simulink model "sim_dist_pos_obs_paper"  (R2020a)
settings: Solver=ode4  StartTime=0.0  StopTime=30.0  FixedStep=0.01  RelTol=1e-3
values from neighbouring files (symbols this model uses):
  alfa_theta = 20    [draw_compare_dist_pos_obs.m]
  alfa_theta_obs = 100    [draw_compare_dist_pos_obs.m]
  beta1 = 1.2    [draw_compare_dist_pos_obs.m]
  beta2 = 0.8    [draw_compare_dist_pos_obs.m]
  c1_diff_sigma_bar_v = diag([25; 30; 20])    [draw_compare_dist_pos_obs.m]
  c1v = diag([16.0; 16.0; 16.0])    [draw_compare_dist_pos_obs.m]
  c2_diff_sigma_bar_v = diag([50; 50; 10])    [draw_compare_dist_pos_obs.m]
  c2v = diag([16.0; 16.0; 16.0])    [draw_compare_dist_pos_obs.m]
  c3_diff_sigma_bar_v = diag([15; 15; 10])    [draw_compare_dist_pos_obs.m]
  c3v = diag([16.0; 16.0; 16.0])    [draw_compare_dist_pos_obs.m]
  delta_p_i_0 = zeros(3, NF)    [draw_compare_dist_pos_obs.m]
  delta_v_i_0 = zeros(3, NF)    [draw_compare_dist_pos_obs.m]
  dp_aa_t = 0.2 * ones(3, 5) + ( 1.0 - 0.2 ) * rand(3, 5)    [draw_compare_dist_pos_obs.m]
  dp_ff_t = [ 0.4 * ones(1, 5) + ( 1.0 - 0.4 ) * rand(1, 5);                      0.4 * ones(1, 5) + ( 1.0 - 0.4 ) * rand(1, 5);                      0.2 * ones(1, 5) + ( 0.6 - 0.2 ) * rand(1, 5) ]    [draw_compare_dist_pos_obs.m]
  dp_phi_t = ( - pi / 2 ) * ones(3, 5) + ( pi / 2 - ( - pi / 2 ) ) * rand(3, 5)    [draw_compare_dist_pos_obs.m]
  etai_0 = zeros(3,5)    [draw_compare_dist_pos_obs.m]
  kai_1_t = 0.02    [draw_compare_dist_pos_obs.m]
  kai_3_t = 0.1    [draw_compare_dist_pos_obs.m]
  kai_chi_1 = diag([6; 6; 6])    [draw_compare_dist_pos_obs.m]
  kai_chi_2 = diag([6; 6; 6])    [draw_compare_dist_pos_obs.m]
  kai_u_1 = diag([8; 8; 8])    [draw_compare_dist_pos_obs.m]
  kai_u_2 = diag([8; 8; 8])    [draw_compare_dist_pos_obs.m]
  ksii_0 = zeros(3,5)    [draw_compare_dist_pos_obs.m]
  l1v = diag([20; 20; 20])    [draw_compare_dist_pos_obs.m]
  l2v = diag([30; 30; 30])    [draw_compare_dist_pos_obs.m]
  Lamd_diff_sigma_bar_v = 0.5    [draw_compare_dist_pos_obs.m]
  mass_i = zeros(1,NF)    [draw_compare_dist_pos_obs.m]
  Mii = diag([1;0;0;0;1])    [draw_compare_dist_pos_obs.m]
  pos0 = zeros(3, 1)    [draw_compare_dist_pos_obs.m]
  PZ0 = P0(3)    [draw_compare_dist_pos_obs.m]
  PZ1 = 10    [draw_compare_dist_pos_obs.m]
  Qci_init = repmat([1;0;0;0],1,NF)    [draw_compare_dist_pos_obs.m]
  R0 = 4    [draw_compare_dist_pos_obs.m]
  R1 = 8    [draw_compare_dist_pos_obs.m]
  Rx2 = 10    [draw_compare_dist_pos_obs.m]
  Ry2 = 6    [draw_compare_dist_pos_obs.m]
  Rz2 = 4    [draw_compare_dist_pos_obs.m]
  T0 = 0    [draw_compare_dist_pos_obs.m]
  T1 = tseq1    (= 10)    [draw_compare_dist_pos_obs.m]
  T12 = tseq1 + tseq12    (= 20)    [draw_compare_dist_pos_obs.m]
  T2 = tseq1 + tseq12 + tseq2    (= 30)    [draw_compare_dist_pos_obs.m]
  theta0 = ( 2 / 5 ) * pi    (= 1.25663706144)    [draw_compare_dist_pos_obs.m]
  vel0 = zeros(3, 1)    [draw_compare_dist_pos_obs.m]
  Wij = [0,0,1,0,0;              0,0,1,1,0;              1,0,0,0,1;              0,1,1,0,0;              0,0,1,0,0]    [draw_compare_dist_pos_obs.m]
  X1 = 8    [draw_compare_dist_pos_obs.m]
  X2 = 2    [draw_compare_dist_pos_obs.m]
  X3 = 3    [draw_compare_dist_pos_obs.m]
  Y1 = 10    [draw_compare_dist_pos_obs.m]
  Y2 = 2    [draw_compare_dist_pos_obs.m]
  Y3 = 4    [draw_compare_dist_pos_obs.m]
  Z1 = 4    [draw_compare_dist_pos_obs.m]
  Z2 = -6    [draw_compare_dist_pos_obs.m]
  Z3 = 2    [draw_compare_dist_pos_obs.m]
  zeta_diff_sigma_bar_v = 0.08    [draw_compare_dist_pos_obs.m]
undefined symbols (not defined in the file or in its folder): cal_frac_squ, p_alfav1, p_alfav2, p_beta1, p_beta2, p_dbeta1, p_dbeta2, p_gamma1_pos, p_gamma1_vel, p_gamma2_pos, p_gamma2_vel, q_alfav1, q_alfav2, q_beta1, q_beta2, q_dbeta1, q_dbeta2, q_gamma1_pos, q_gamma1_vel, q_gamma2_pos, q_gamma2_vel
(part 3 of 5)

== matlab function sim_dist_pos_obs_paper/combine translational disturbance ==
  data: dp_vec output; dp_1 input; dp_2 input; dp_3 input; dp_4 input; dp_5 input
function dp_vec = fcn(dp_1, dp_2, dp_3, dp_4, dp_5)
%%%% 合并领导者编队跟踪误差结果
dp_vec = [dp_1(:), dp_2(:), dp_3(:), dp_4(:), dp_5(:)];

== matlab function sim_dist_pos_obs_paper/cal differentiator d_sigma_bar_v_hat agent 2/trans to column23 ==
  data: x input; y output
function y = fcn(x)
y = x(:);

== matlab function sim_dist_pos_obs_paper/cal differentiator d_sigma_bar_v_hat agent 2/trans to column24 ==
  data: x input; y output
function y = fcn(x)
y = x(:);

== matlab function sim_dist_pos_obs_paper/cal differentiator d_sigma_bar_v_hat agent 2/trans to column25 ==
  data: x input; y output
function y = fcn(x)
y = x(:);

== matlab function sim_dist_pos_obs_paper/cal differentiator d_sigma_bar_v_hat agent 3/cal differentiator ==
  data: c1 input; d_sigma_bar_v_hat output; d_dsigma_bar_v_hat output; d_d2sigma_bar_v_hat output; c2 input; c3 input; chi_t input; sigma_bar_v_sig_1 input; sigma_bar_v_sig_2 input; sigma_bar_v_sig_3 input; sigma_bar_v_sig_4 input; sigma_bar_v_sig_5 input; sigma_bar_v_sig_6 input; d_sigma_bar_v_hat input; d2_sigma_bar_v_hat input
function [d_sigma_bar_v_hat, d_dsigma_bar_v_hat, d_d2sigma_bar_v_hat] = fcn(c1, c2, c3, chi_t, sigma_bar_v_sig_1, sigma_bar_v_sig_2, sigma_bar_v_sig_3, ...
                                                                                                                                                sigma_bar_v_sig_4, sigma_bar_v_sig_5, sigma_bar_v_sig_6, d_sigma_bar_v_hat, d2_sigma_bar_v_hat)
d_d2sigma_bar_v_hat = -chi_t .* c1 * sigma_bar_v_sig_1(:) - (1 - chi_t) .* c1 * sigma_bar_v_sig_2(:);
d_dsigma_bar_v_hat = -chi_t .* c2 * sigma_bar_v_sig_3(:) - (1 - chi_t) .* c2 * sigma_bar_v_sig_4(:) + d2_sigma_bar_v_hat(:);
d_sigma_bar_v_hat = -chi_t .* c3 * sigma_bar_v_sig_5(:) - (1 - chi_t) .* c3 * sigma_bar_v_sig_6(:) + d_sigma_bar_v_hat(:);

== matlab function sim_dist_pos_obs_paper/cal differentiator d_sigma_bar_v_hat agent 3/cal sig ==
  data: x input; z output; y input
function z = fcn(x, y)
z = x(:) .* sign(y(:));

== matlab function sim_dist_pos_obs_paper/depart Re5 ==
  data: y output; x input
function y = fcn(x)
y = x(:,:,5);

end

== matlab function sim_dist_pos_obs_paper/depart Re1 ==
  data: y output; x input
function y = fcn(x)
y = x(:,:,1);

end

== matlab function sim_dist_pos_obs_paper/depart Re2 ==
  data: y output; x input
function y = fcn(x)
y = x(:,:,2);

end

== matlab function sim_dist_pos_obs_paper/depart Re3 ==
  data: y output; x input
function y = fcn(x)
y = x(:,:,3);

end

== matlab function sim_dist_pos_obs_paper/depart Re4 ==
  data: y output; x input
function y = fcn(x)
y = x(:,:,4);

end

== matlab function sim_dist_pos_obs_paper/cal differentiator d_sigma_bar_v_hat agent 3/cal sig1 ==
  data: x input; z output; y input
function z = fcn(x, y)
z = x(:) .* sign(y(:));

== matlab function sim_dist_pos_obs_paper/cal differentiator d_sigma_bar_v_hat agent 3/cal sig2 ==
  data: x input; z output; y input
function z = fcn(x, y)
z = x(:) .* sign(y(:));

== matlab function sim_dist_pos_obs_paper/cal differentiator d_sigma_bar_v_hat agent 3/cal sig3 ==
  data: x input; z output; y input
function z = fcn(x, y)
z = x(:) .* sign(y(:));

== matlab function sim_dist_pos_obs_paper/cal abs 2 ==
  data: x input; y output
function y = fcn(x)
y = abs(x(:));

== matlab function sim_dist_pos_obs_paper/cal differentiator d_sigma_bar_v_hat agent 3/cal sig4 ==
  data: x input; z output; y input
function z = fcn(x, y)
z = x(:) .* sign(y(:));

== matlab function sim_dist_pos_obs_paper/cal differentiator d_sigma_bar_v_hat agent 3/cal sig5 ==
  data: x input; z output; y input
function z = fcn(x, y)
z = x(:) .* sign(y(:));

== matlab function sim_dist_pos_obs_paper/choose ksi_est_err 1 ==
  data: x input; y output
function y = fcn(x)
iiuav = 1;
y = x(:,iiuav);

== matlab function sim_dist_pos_obs_paper/trans to column35 ==
  data: x input; y output
function y = fcn(x)
y = x(:);

== matlab function sim_dist_pos_obs_paper/cal differentiator d_sigma_bar_v_hat agent 3/choose sigma_bar_v ==
  data: x input; y output
function y = fcn(x)
iiuav = 3;
y = x(:,iiuav);

== matlab function sim_dist_pos_obs_paper/cal differentiator d_sigma_bar_v_hat agent 3/trans to column20 ==
  data: x input; y output
function y = fcn(x)
y = x(:);

== matlab function sim_dist_pos_obs_paper/cal differentiator d_sigma_bar_v_hat agent 3/trans to column21 ==
  data: x input; y output
function y = fcn(x)
y = x(:);

== matlab function sim_dist_pos_obs_paper/cal differentiator d_sigma_bar_v_hat agent 3/trans to column22 ==
  data: x input; y output
function y = fcn(x)
y = x(:);

== matlab function sim_dist_pos_obs_paper/cal differentiator d_sigma_bar_v_hat agent 3/trans to column23 ==
  data: x input; y output
function y = fcn(x)
y = x(:);

== matlab function sim_dist_pos_obs_paper/cal differentiator d_sigma_bar_v_hat agent 3/trans to column24 ==
  data: x input; y output
function y = fcn(x)
y = x(:);

== matlab function sim_dist_pos_obs_paper/cal theta_err_ksi agent 1 ==
  data: alfa_theta input; err_ksi_squ_1_node_1 input; theta_err_ksi_1_1 output; err_ksi_squ_2_node_1 input; err_ksi_vec input; theta_err_ksi_2_1 output
function [theta_err_ksi_1_1, theta_err_ksi_2_1] = fcn(alfa_theta, err_ksi_squ_1_node_1, err_ksi_squ_2_node_1, err_ksi_vec)
%%%% 计算平滑递增函数
iiuav = 1;
theta_err_ksi_1_1 = err_ksi_squ_1_node_1(:) .* ( -1 + 2 ./ ( 1 + exp( -alfa_theta .* err_ksi_vec(:,iiuav) ) ) );
theta_err_ksi_2_1 = err_ksi_squ_2_node_1(:) .* ( -1 + 2 ./ ( 1 + exp( -alfa_theta .* err_ksi_vec(:,iiuav) ) ) );

== matlab function sim_dist_pos_obs_paper/cal differentiator d_sigma_bar_v_hat agent 3/trans to column25 ==
  data: x input; y output
function y = fcn(x)
y = x(:);

== matlab function sim_dist_pos_obs_paper/cal differentiator d_sigma_bar_v_hat agent 4/cal differentiator ==
  data: c1 input; d_sigma_bar_v_hat output; d_dsigma_bar_v_hat output; d_d2sigma_bar_v_hat output; c2 input; c3 input; chi_t input; sigma_bar_v_sig_1 input; sigma_bar_v_sig_2 input; sigma_bar_v_sig_3 input; sigma_bar_v_sig_4 input; sigma_bar_v_sig_5 input; sigma_bar_v_sig_6 input; d_sigma_bar_v_hat input; d2_sigma_bar_v_hat input
function [d_sigma_bar_v_hat, d_dsigma_bar_v_hat, d_d2sigma_bar_v_hat] = fcn(c1, c2, c3, chi_t, sigma_bar_v_sig_1, sigma_bar_v_sig_2, sigma_bar_v_sig_3, ...
                                                                                                                                                sigma_bar_v_sig_4, sigma_bar_v_sig_5, sigma_bar_v_sig_6, d_sigma_bar_v_hat, d2_sigma_bar_v_hat)
d_d2sigma_bar_v_hat = -chi_t .* c1 * sigma_bar_v_sig_1(:) - (1 - chi_t) .* c1 * sigma_bar_v_sig_2(:);
d_dsigma_bar_v_hat = -chi_t .* c2 * sigma_bar_v_sig_3(:) - (1 - chi_t) .* c2 * sigma_bar_v_sig_4(:) + d2_sigma_bar_v_hat(:);
d_sigma_bar_v_hat = -chi_t .* c3 * sigma_bar_v_sig_5(:) - (1 - chi_t) .* c3 * sigma_bar_v_sig_6(:) + d_sigma_bar_v_hat(:);

== matlab function sim_dist_pos_obs_paper/cal differentiator d_sigma_bar_v_hat agent 4/cal sig ==
  data: x input; z output; y input
function z = fcn(x, y)
z = x(:) .* sign(y(:));

== matlab function sim_dist_pos_obs_paper/cal differentiator d_sigma_bar_v_hat agent 4/cal sig1 ==
  data: x input; z output; y input
function z = fcn(x, y)
z = x(:) .* sign(y(:));

== matlab function sim_dist_pos_obs_paper/cal differentiator d_sigma_bar_v_hat agent 4/cal sig2 ==
  data: x input; z output; y input
function z = fcn(x, y)
z = x(:) .* sign(y(:));

== matlab function sim_dist_pos_obs_paper/cal differentiator d_sigma_bar_v_hat agent 4/cal sig3 ==
  data: x input; z output; y input
function z = fcn(x, y)
z = x(:) .* sign(y(:));

== matlab function sim_dist_pos_obs_paper/cal differentiator d_sigma_bar_v_hat agent 4/cal sig4 ==
  data: x input; z output; y input
function z = fcn(x, y)
z = x(:) .* sign(y(:));

== matlab function sim_dist_pos_obs_paper/cal differentiator d_sigma_bar_v_hat agent 4/cal sig5 ==
  data: x input; z output; y input
function z = fcn(x, y)
z = x(:) .* sign(y(:));

== matlab function sim_dist_pos_obs_paper/cal differentiator d_sigma_bar_v_hat agent 4/choose sigma_bar_v ==
  data: x input; y output
function y = fcn(x)
iiuav = 4;
y = x(:,iiuav);

== matlab function sim_dist_pos_obs_paper/cal differentiator d_sigma_bar_v_hat agent 4/trans to column20 ==
  data: x input; y output
function y = fcn(x)
y = x(:);

== matlab function sim_dist_pos_obs_paper/cal differentiator d_sigma_bar_v_hat agent 4/trans to column21 ==
  data: x input; y output
function y = fcn(x)
y = x(:);

== matlab function sim_dist_pos_obs_paper/cal differentiator d_sigma_bar_v_hat agent 4/trans to column22 ==
  data: x input; y output
function y = fcn(x)
y = x(:);

== matlab function sim_dist_pos_obs_paper/cal differentiator d_sigma_bar_v_hat agent 4/trans to column23 ==
  data: x input; y output
function y = fcn(x)
y = x(:);

== matlab function sim_dist_pos_obs_paper/trans to column1 ==
  data: x input; y output
function y = fcn(x)
y = x(:);

== matlab function sim_dist_pos_obs_paper/cal Rci from ui ==
  data: Rci output; mi input; ui input
function Rci = fcn(mi, ui)
Rci = zeros(3,3,5);
for iiuav = 1:5
    Rci(:,:,iiuav) = cal_Rc_with_u(mi(iiuav), ui(:,iiuav));
end

end

== matlab function sim_dist_pos_obs_paper/cal differentiator d_sigma_bar_v_hat agent 4/trans to column24 ==
  data: x input; y output
function y = fcn(x)
y = x(:);

== matlab function sim_dist_pos_obs_paper/cal differentiator d_sigma_bar_v_hat agent 4/trans to column25 ==
  data: x input; y output
function y = fcn(x)
y = x(:);

== matlab function sim_dist_pos_obs_paper/cal differentiator d_sigma_bar_v_hat agent 5/cal differentiator ==
  data: c1 input; d_sigma_bar_v_hat output; d_dsigma_bar_v_hat output; d_d2sigma_bar_v_hat output; c2 input; c3 input; chi_t input; sigma_bar_v_sig_1 input; sigma_bar_v_sig_2 input; sigma_bar_v_sig_3 input; sigma_bar_v_sig_4 input; sigma_bar_v_sig_5 input; sigma_bar_v_sig_6 input; d_sigma_bar_v_hat input; d2_sigma_bar_v_hat input
function [d_sigma_bar_v_hat, d_dsigma_bar_v_hat, d_d2sigma_bar_v_hat] = fcn(c1, c2, c3, chi_t, sigma_bar_v_sig_1, sigma_bar_v_sig_2, sigma_bar_v_sig_3, ...
                                                                                                                                                sigma_bar_v_sig_4, sigma_bar_v_sig_5, sigma_bar_v_sig_6, d_sigma_bar_v_hat, d2_sigma_bar_v_hat)
d_d2sigma_bar_v_hat = -chi_t .* c1 * sigma_bar_v_sig_1(:) - (1 - chi_t) .* c1 * sigma_bar_v_sig_2(:);
d_dsigma_bar_v_hat = -chi_t .* c2 * sigma_bar_v_sig_3(:) - (1 - chi_t) .* c2 * sigma_bar_v_sig_4(:) + d2_sigma_bar_v_hat(:);
d_sigma_bar_v_hat = -chi_t .* c3 * sigma_bar_v_sig_5(:) - (1 - chi_t) .* c3 * sigma_bar_v_sig_6(:) + d_sigma_bar_v_hat(:);

== matlab function sim_dist_pos_obs_paper/cal differentiator d_sigma_bar_v_hat agent 5/cal sig ==
  data: x input; z output; y input
function z = fcn(x, y)
z = x(:) .* sign(y(:));

== matlab function sim_dist_pos_obs_paper/cal differentiator d_sigma_bar_v_hat agent 5/cal sig1 ==
  data: x input; z output; y input
function z = fcn(x, y)
z = x(:) .* sign(y(:));

== matlab function sim_dist_pos_obs_paper/cal differentiator d_sigma_bar_v_hat agent 5/cal sig2 ==
  data: x input; z output; y input
function z = fcn(x, y)
z = x(:) .* sign(y(:));

== matlab function sim_dist_pos_obs_paper/cal differentiator d_sigma_bar_v_hat agent 5/cal sig3 ==
  data: x input; z output; y input
function z = fcn(x, y)
z = x(:) .* sign(y(:));

== matlab function sim_dist_pos_obs_paper/cal abs 3 ==
  data: x input; y output
function y = fcn(x)
y = abs(x(:));

== matlab function sim_dist_pos_obs_paper/cal differentiator d_sigma_bar_v_hat agent 5/cal sig4 ==
  data: x input; z output; y input
function z = fcn(x, y)
z = x(:) .* sign(y(:));

== matlab function sim_dist_pos_obs_paper/cal differentiator d_sigma_bar_v_hat agent 5/cal sig5 ==
  data: x input; z output; y input
function z = fcn(x, y)
z = x(:) .* sign(y(:));

== matlab function sim_dist_pos_obs_paper/cal differentiator d_sigma_bar_v_hat agent 5/choose sigma_bar_v ==
  data: x input; y output
function y = fcn(x)
iiuav = 5;
y = x(:,iiuav);

== matlab function sim_dist_pos_obs_paper/cal differentiator d_sigma_bar_v_hat agent 5/trans to column20 ==
  data: x input; y output
function y = fcn(x)
y = x(:);

== matlab function sim_dist_pos_obs_paper/cal differentiator d_sigma_bar_v_hat agent 5/trans to column21 ==
  data: x input; y output
function y = fcn(x)
y = x(:);

== matlab function sim_dist_pos_obs_paper/cal differentiator d_sigma_bar_v_hat agent 5/trans to column22 ==
  data: x input; y output
function y = fcn(x)
y = x(:);

== matlab function sim_dist_pos_obs_paper/cal differentiator d_sigma_bar_v_hat agent 5/trans to column23 ==
  data: x input; y output
function y = fcn(x)
y = x(:);

== matlab function sim_dist_pos_obs_paper/cal differentiator d_sigma_bar_v_hat agent 5/trans to column24 ==
  data: x input; y output
function y = fcn(x)
y = x(:);

== matlab function sim_dist_pos_obs_paper/cal differentiator d_sigma_bar_v_hat agent 5/trans to column25 ==
  data: x input; y output
function y = fcn(x)
y = x(:);

== matlab function sim_dist_pos_obs_paper/cal abs 4 ==
  data: x input; y output
function y = fcn(x)
y = abs(x(:));

== matlab function sim_dist_pos_obs_paper/combine d_sigma_bar_v_est ==
  data: d_sigma_bar_v_est_1 input; d_sigma_bar_v_est_2 input; d_sigma_bar_v_est_3 input; d_sigma_bar_v_est_4 input; d_sigma_bar_v_est_5 input; d_sigma_bar_v_vec output
function d_sigma_bar_v_vec  = fcn(d_sigma_bar_v_est_1, d_sigma_bar_v_est_2, d_sigma_bar_v_est_3, d_sigma_bar_v_est_4, d_sigma_bar_v_est_5)
%%%% 合并用微分器求得的虚拟速度控制量导数
d_sigma_bar_v_vec = [d_sigma_bar_v_est_1(:), d_sigma_bar_v_est_2(:), d_sigma_bar_v_est_3(:), d_sigma_bar_v_est_4(:), d_sigma_bar_v_est_5(:)];

== matlab function sim_dist_pos_obs_paper/cal abs 21 ==
  data: x input; y output
function y = fcn(x)
y = abs(x(:));

== matlab function sim_dist_pos_obs_paper/cal abs 22 ==
  data: x input; y output
function y = fcn(x)
y = abs(x(:));

== matlab function sim_dist_pos_obs_paper/choose ksi_est_err 21 ==
  data: x input; y output
function y = fcn(x)
iiuav = 1;
y = x(:,iiuav);

== matlab function sim_dist_pos_obs_paper/choose ksi_est_err 22 ==
  data: x input; y output
function y = fcn(x)
iiuav = 1;
y = x(:,iiuav);

== matlab function sim_dist_pos_obs_paper/trans to column20 ==
  data: x input; y output
function y = fcn(x)
y = x(:);

== matlab function sim_dist_pos_obs_paper/trans to column21 ==
  data: x input; y output
function y = fcn(x)
y = x(:);

== matlab function sim_dist_pos_obs_paper/cal theta_sigma_bar_v_tilt agent 1 ==
  data: alfa_theta input; sigma_bar_v_tilt_squ_1_1 input; theta_sigma_bar_v_tilt_1_1 output; sigma_bar_v_tilt_squ_2_1 input; sigma_bar_v_tilt_vec input; theta_sigma_bar_v_tilt_2_1 output
function [theta_sigma_bar_v_tilt_1_1, theta_sigma_bar_v_tilt_2_1] = fcn(alfa_theta, sigma_bar_v_tilt_squ_1_1, sigma_bar_v_tilt_squ_2_1, sigma_bar_v_tilt_vec)
%%%% 计算平滑递增函数
iiuav = 1;
theta_sigma_bar_v_tilt_1_1 = sigma_bar_v_tilt_squ_1_1(:) .* ( -1 + 2 ./ ( 1 + exp( -alfa_theta .* sigma_bar_v_tilt_vec(:,iiuav) ) ) );
theta_sigma_bar_v_tilt_2_1 = sigma_bar_v_tilt_squ_2_1(:) .* ( -1 + 2 ./ ( 1 + exp( -alfa_theta .* sigma_bar_v_tilt_vec(:,iiuav) ) ) );

== matlab function sim_dist_pos_obs_paper/cal abs 23 ==
  data: x input; y output
function y = fcn(x)
y = abs(x(:));

== matlab function sim_dist_pos_obs_paper/cal theta_err_ksi agent 2 ==
  data: alfa_theta input; err_ksi_squ_1_node_2 input; theta_err_ksi_1_2 output; err_ksi_squ_2_node_2 input; err_ksi_vec input; theta_err_ksi_2_2 output
function [theta_err_ksi_1_2, theta_err_ksi_2_2] = fcn(alfa_theta, err_ksi_squ_1_node_2, err_ksi_squ_2_node_2, err_ksi_vec)
%%%% 计算平滑递增函数
iiuav = 2;
theta_err_ksi_1_2 = err_ksi_squ_1_node_2(:) .* ( -1 + 2 ./ ( 1 + exp( -alfa_theta .* err_ksi_vec(:,iiuav) ) ) );
theta_err_ksi_2_2 = err_ksi_squ_2_node_2(:) .* ( -1 + 2 ./ ( 1 + exp( -alfa_theta .* err_ksi_vec(:,iiuav) ) ) );

== matlab function sim_dist_pos_obs_paper/cal abs 24 ==
  data: x input; y output
function y = fcn(x)
y = abs(x(:));

== matlab function sim_dist_pos_obs_paper/cal theta_sigma_bar_v_tilt agent 2 ==
  data: alfa_theta input; sigma_bar_v_tilt_squ_1_2 input; theta_sigma_bar_v_tilt_1_2 output; sigma_bar_v_tilt_squ_2_2 input; sigma_bar_v_tilt_vec input; theta_sigma_bar_v_tilt_2_2 output
function [theta_sigma_bar_v_tilt_1_2, theta_sigma_bar_v_tilt_2_2] = fcn(alfa_theta, sigma_bar_v_tilt_squ_1_2, sigma_bar_v_tilt_squ_2_2, sigma_bar_v_tilt_vec)
%%%% 计算平滑递增函数
iiuav = 2;
theta_sigma_bar_v_tilt_1_2 = sigma_bar_v_tilt_squ_1_2(:) .* ( -1 + 2 ./ ( 1 + exp( -alfa_theta .* sigma_bar_v_tilt_vec(:,iiuav) ) ) );
theta_sigma_bar_v_tilt_2_2 = sigma_bar_v_tilt_squ_2_2(:) .* ( -1 + 2 ./ ( 1 + exp( -alfa_theta .* sigma_bar_v_tilt_vec(:,iiuav) ) ) );

== matlab function sim_dist_pos_obs_paper/choose ksi_est_err 23 ==
  data: x input; y output
function y = fcn(x)
iiuav = 2;
y = x(:,iiuav);

== matlab function sim_dist_pos_obs_paper/choose ksi_est_err 24 ==
  data: x input; y output
function y = fcn(x)
iiuav = 2;
y = x(:,iiuav);

== matlab function sim_dist_pos_obs_paper/trans to column22 ==
  data: x input; y output
function y = fcn(x)
y = x(:);

== matlab function sim_dist_pos_obs_paper/trans to column23 ==
  data: x input; y output
function y = fcn(x)
y = x(:);

== matlab function sim_dist_pos_obs_paper/cal abs 25 ==
  data: x input; y output
function y = fcn(x)
y = abs(x(:));

== matlab function sim_dist_pos_obs_paper/cal abs 26 ==
  data: x input; y output
function y = fcn(x)
y = abs(x(:));

== matlab function sim_dist_pos_obs_paper/cal theta_sigma_bar_v_tilt agent 3 ==
  data: alfa_theta input; sigma_bar_v_tilt_squ_1_3 input; theta_sigma_bar_v_tilt_1_3 output; sigma_bar_v_tilt_squ_2_3 input; sigma_bar_v_tilt_vec input; theta_sigma_bar_v_tilt_2_3 output
function [theta_sigma_bar_v_tilt_1_3, theta_sigma_bar_v_tilt_2_3] = fcn(alfa_theta, sigma_bar_v_tilt_squ_1_3, sigma_bar_v_tilt_squ_2_3, sigma_bar_v_tilt_vec)
%%%% 计算平滑递增函数
iiuav = 3;
theta_sigma_bar_v_tilt_1_3 = sigma_bar_v_tilt_squ_1_3(:) .* ( -1 + 2 ./ ( 1 + exp( -alfa_theta .* sigma_bar_v_tilt_vec(:,iiuav) ) ) );
theta_sigma_bar_v_tilt_2_3 = sigma_bar_v_tilt_squ_2_3(:) .* ( -1 + 2 ./ ( 1 + exp( -alfa_theta .* sigma_bar_v_tilt_vec(:,iiuav) ) ) );

== matlab function sim_dist_pos_obs_paper/choose ksi_est_err 25 ==
  data: x input; y output
function y = fcn(x)
iiuav = 3;
y = x(:,iiuav);

== matlab function sim_dist_pos_obs_paper/choose ksi_est_err 26 ==
  data: x input; y output
function y = fcn(x)
iiuav = 3;
y = x(:,iiuav);

== matlab function sim_dist_pos_obs_paper/trans to column24 ==
  data: x input; y output
function y = fcn(x)
y = x(:);

== matlab function sim_dist_pos_obs_paper/trans to column25 ==
  data: x input; y output
function y = fcn(x)
y = x(:);

== matlab function sim_dist_pos_obs_paper/cal abs 27 ==
  data: x input; y output
function y = fcn(x)
y = abs(x(:));

== matlab function sim_dist_pos_obs_paper/cal abs 28 ==
  data: x input; y output
function y = fcn(x)
y = abs(x(:));

== matlab function sim_dist_pos_obs_paper/choose ksi_est_err 3 ==
  data: x input; y output
function y = fcn(x)
iiuav = 2;
y = x(:,iiuav);

== matlab function sim_dist_pos_obs_paper/cal theta_sigma_bar_v_tilt agent 4 ==
  data: alfa_theta input; sigma_bar_v_tilt_squ_1_4 input; theta_sigma_bar_v_tilt_1_4 output; sigma_bar_v_tilt_squ_2_4 input; sigma_bar_v_tilt_vec input; theta_sigma_bar_v_tilt_2_4 output
function [theta_sigma_bar_v_tilt_1_4, theta_sigma_bar_v_tilt_2_4] = fcn(alfa_theta, sigma_bar_v_tilt_squ_1_4, sigma_bar_v_tilt_squ_2_4, sigma_bar_v_tilt_vec)
%%%% 计算平滑递增函数
iiuav = 4;
theta_sigma_bar_v_tilt_1_4 = sigma_bar_v_tilt_squ_1_4(:) .* ( -1 + 2 ./ ( 1 + exp( -alfa_theta .* sigma_bar_v_tilt_vec(:,iiuav) ) ) );
theta_sigma_bar_v_tilt_2_4 = sigma_bar_v_tilt_squ_2_4(:) .* ( -1 + 2 ./ ( 1 + exp( -alfa_theta .* sigma_bar_v_tilt_vec(:,iiuav) ) ) );

== matlab function sim_dist_pos_obs_paper/choose ksi_est_err 27 ==
  data: x input; y output
function y = fcn(x)
iiuav = 4;
y = x(:,iiuav);

== matlab function sim_dist_pos_obs_paper/choose ksi_est_err 28 ==
  data: x input; y output
function y = fcn(x)
iiuav = 4;
y = x(:,iiuav);

== matlab function sim_dist_pos_obs_paper/trans to column26 ==
  data: x input; y output
function y = fcn(x)
y = x(:);

== matlab function sim_dist_pos_obs_paper/trans to column27 ==
  data: x input; y output
function y = fcn(x)
y = x(:);

== matlab function sim_dist_pos_obs_paper/cal abs 29 ==
  data: x input; y output
function y = fcn(x)
y = abs(x(:));

== matlab function sim_dist_pos_obs_paper/cal abs 30 ==
  data: x input; y output
function y = fcn(x)
y = abs(x(:));

== matlab function sim_dist_pos_obs_paper/cal theta_sigma_bar_v_tilt agent 5 ==
  data: alfa_theta input; sigma_bar_v_tilt_squ_1_5 input; theta_sigma_bar_v_tilt_1_5 output; sigma_bar_v_tilt_squ_2_5 input; sigma_bar_v_tilt_vec input; theta_sigma_bar_v_tilt_2_5 output
function [theta_sigma_bar_v_tilt_1_5, theta_sigma_bar_v_tilt_2_5] = fcn(alfa_theta, sigma_bar_v_tilt_squ_1_5, sigma_bar_v_tilt_squ_2_5, sigma_bar_v_tilt_vec)
%%%% 计算平滑递增函数
iiuav = 5;
theta_sigma_bar_v_tilt_1_5 = sigma_bar_v_tilt_squ_1_5(:) .* ( -1 + 2 ./ ( 1 + exp( -alfa_theta .* sigma_bar_v_tilt_vec(:,iiuav) ) ) );
theta_sigma_bar_v_tilt_2_5 = sigma_bar_v_tilt_squ_2_5(:) .* ( -1 + 2 ./ ( 1 + exp( -alfa_theta .* sigma_bar_v_tilt_vec(:,iiuav) ) ) );

== matlab function sim_dist_pos_obs_paper/choose ksi_est_err 29 ==
  data: x input; y output
function y = fcn(x)
iiuav = 5;
y = x(:,iiuav);

== matlab function sim_dist_pos_obs_paper/choose ksi_est_err 4 ==
  data: x input; y output
function y = fcn(x)
iiuav = 2;
y = x(:,iiuav);

== matlab function sim_dist_pos_obs_paper/choose ksi_est_err 30 ==
  data: x input; y output
function y = fcn(x)
iiuav = 5;
y = x(:,iiuav);

== matlab function sim_dist_pos_obs_paper/trans to column28 ==
  data: x input; y output
function y = fcn(x)
y = x(:);

== matlab function sim_dist_pos_obs_paper/trans to column29 ==
  data: x input; y output
function y = fcn(x)
y = x(:);

== matlab function sim_dist_pos_obs_paper/combine theta_sigma_bar_v_tilt ==
  data: theta_sigma_bar_v_tilt_1_1 input; theta_sigma_bar_v_tilt_1_2 input; theta_sigma_bar_v_tilt_1_3 input; theta_sigma_bar_v_tilt_1_4 input; theta_sigma_bar_v_tilt_1_5 input; theta_sigma_bar_v_tilt_1_vec output; theta_sigma_bar_v_tilt_2_1 input; theta_sigma_bar_v_tilt_2_vec output; theta_sigma_bar_v_tilt_2_2 input; theta_sigma_bar_v_tilt_2_3 input; theta_sigma_bar_v_tilt_2_4 input; theta_sigma_bar_v_tilt_2_5 input
function [theta_sigma_bar_v_tilt_1_vec, theta_sigma_bar_v_tilt_2_vec]  = fcn(theta_sigma_bar_v_tilt_1_1, theta_sigma_bar_v_tilt_1_2, theta_sigma_bar_v_tilt_1_3, theta_sigma_bar_v_tilt_1_4, theta_sigma_bar_v_tilt_1_5, ...
                                                                                                                                            theta_sigma_bar_v_tilt_2_1, theta_sigma_bar_v_tilt_2_2, theta_sigma_bar_v_tilt_2_3, theta_sigma_bar_v_tilt_2_4, theta_sigma_bar_v_tilt_2_5)
%%%% 合并领导者位置观测器输出结果
theta_sigma_bar_v_tilt_1_vec = [theta_sigma_bar_v_tilt_1_1(:), theta_sigma_bar_v_tilt_1_2(:), theta_sigma_bar_v_tilt_1_3(:), theta_sigma_bar_v_tilt_1_4(:), theta_sigma_bar_v_tilt_1_5(:)];
theta_sigma_bar_v_tilt_2_vec = [theta_sigma_bar_v_tilt_2_1(:), theta_sigma_bar_v_tilt_2_2(:), theta_sigma_bar_v_tilt_2_3(:), theta_sigma_bar_v_tilt_2_4(:), theta_sigma_bar_v_tilt_2_5(:)];

== matlab function sim_dist_pos_obs_paper/cal sigma_bar_v_hat agent 1 ==
  data: c1v input; c2v input; theta_sigma_bar_v_tilt_1_vec input; d_sigma_bar_v_hat_1 output; theta_sigma_bar_v_tilt_2_vec input; d_sigma_bar_v_vec input
function d_sigma_bar_v_hat_1 = fcn(c1v, c2v, theta_sigma_bar_v_tilt_1_vec, theta_sigma_bar_v_tilt_2_vec, d_sigma_bar_v_vec)
%%%% 计算扰动观测器中虚拟速度控制量观测值sigma_v_hat的微分方程
iiuav = 1;
d_sigma_bar_v_hat_1 = d_sigma_bar_v_vec(:,iiuav) + ...
                                            c1v * theta_sigma_bar_v_tilt_1_vec(:,iiuav) + ...
                                            c2v * theta_sigma_bar_v_tilt_2_vec(:,iiuav);

== matlab function sim_dist_pos_obs_paper/cal sigma_bar_v_hat agent 2 ==
  data: c1v input; c2v input; theta_sigma_bar_v_tilt_1_vec input; d_sigma_bar_v_hat_2 output; theta_sigma_bar_v_tilt_2_vec input; d_sigma_bar_v_vec input
function d_sigma_bar_v_hat_2 = fcn(c1v, c2v, theta_sigma_bar_v_tilt_1_vec, theta_sigma_bar_v_tilt_2_vec, d_sigma_bar_v_vec)
%%%% 计算扰动观测器中虚拟速度控制量观测值sigma_v_hat的微分方程
iiuav = 2;
d_sigma_bar_v_hat_2 = d_sigma_bar_v_vec(:,iiuav) + ...
                                            c1v * theta_sigma_bar_v_tilt_1_vec(:,iiuav) + ...
                                            c2v * theta_sigma_bar_v_tilt_2_vec(:,iiuav);

== matlab function sim_dist_pos_obs_paper/cal sigma_bar_v_hat agent 3 ==
  data: c1v input; c2v input; theta_sigma_bar_v_tilt_1_vec input; d_sigma_bar_v_hat_3 output; theta_sigma_bar_v_tilt_2_vec input; d_sigma_bar_v_vec input
function d_sigma_bar_v_hat_3 = fcn(c1v, c2v, theta_sigma_bar_v_tilt_1_vec, theta_sigma_bar_v_tilt_2_vec, d_sigma_bar_v_vec)
%%%% 计算扰动观测器中虚拟速度控制量观测值sigma_v_hat的微分方程
iiuav = 3;
d_sigma_bar_v_hat_3 = d_sigma_bar_v_vec(:,iiuav) + ...
                                            c1v * theta_sigma_bar_v_tilt_1_vec(:,iiuav) + ...
                                            c2v * theta_sigma_bar_v_tilt_2_vec(:,iiuav);

== matlab function sim_dist_pos_obs_paper/trans to column2 ==
  data: x input; y output
function y = fcn(x)
y = x(:);

== matlab function sim_dist_pos_obs_paper/cal sigma_bar_v_hat agent 4 ==
  data: c1v input; c2v input; theta_sigma_bar_v_tilt_1_vec input; d_sigma_bar_v_hat_4 output; theta_sigma_bar_v_tilt_2_vec input; d_sigma_bar_v_vec input
function d_sigma_bar_v_hat_4 = fcn(c1v, c2v, theta_sigma_bar_v_tilt_1_vec, theta_sigma_bar_v_tilt_2_vec, d_sigma_bar_v_vec)
%%%% 计算扰动观测器中虚拟速度控制量观测值sigma_v_hat的微分方程
iiuav = 4;
d_sigma_bar_v_hat_4 = d_sigma_bar_v_vec(:,iiuav) + ...
                                            c1v * theta_sigma_bar_v_tilt_1_vec(:,iiuav) + ...
                                            c2v * theta_sigma_bar_v_tilt_2_vec(:,iiuav);

== matlab function sim_dist_pos_obs_paper/cal sigma_bar_v_hat agent 5 ==
  data: c1v input; c2v input; theta_sigma_bar_v_tilt_1_vec input; d_sigma_bar_v_hat_5 output; theta_sigma_bar_v_tilt_2_vec input; d_sigma_bar_v_vec input
function d_sigma_bar_v_hat_5 = fcn(c1v, c2v, theta_sigma_bar_v_tilt_1_vec, theta_sigma_bar_v_tilt_2_vec, d_sigma_bar_v_vec)
%%%% 计算扰动观测器中虚拟速度控制量观测值sigma_v_hat的微分方程
iiuav = 5;
d_sigma_bar_v_hat_5 = d_sigma_bar_v_vec(:,iiuav) + ...
                                            c1v * theta_sigma_bar_v_tilt_1_vec(:,iiuav) + ...
                                            c2v * theta_sigma_bar_v_tilt_2_vec(:,iiuav);

== matlab function sim_dist_pos_obs_paper/cal combine sigma_bar_v_tilt ==
  data: sigma_bar_v_vec input; sigma_bar_v_hat_vec input; sigma_bar_v_tilt_vec output
function sigma_bar_v_tilt_vec = fcn(sigma_bar_v_vec, sigma_bar_v_hat_vec)
%%%% 计算虚拟速度观测误差sigma_bar_v_tilt
sigma_bar_v_tilt_vec = zeros(3,5);
for iiuav = 1:5
    sigma_bar_v_tilt_vec(:,iiuav) = sigma_bar_v_vec(:,iiuav) - sigma_bar_v_hat_vec(:,iiuav);
end

== matlab function sim_dist_pos_obs_paper/combine sigma_bar_v_hat ==
  data: sigma_bar_v_hat_1 input; sigma_bar_v_hat_2 input; sigma_bar_v_hat_3 input; sigma_bar_v_hat_4 input; sigma_bar_v_hat_5 input; sigma_bar_v_hat_vec output
function sigma_bar_v_hat_vec  = fcn(sigma_bar_v_hat_1, sigma_bar_v_hat_2, sigma_bar_v_hat_3, sigma_bar_v_hat_4, sigma_bar_v_hat_5)
%%%% 合并虚拟速度控制量观测值sigma_bar_v_hat
sigma_bar_v_hat_vec = [sigma_bar_v_hat_1(:), sigma_bar_v_hat_2(:), sigma_bar_v_hat_3(:), sigma_bar_v_hat_4(:), sigma_bar_v_hat_5(:)];

== matlab function sim_dist_pos_obs_paper/cal dp_hat agent 1 ==
  data: c3v input; d_sigma_bar_v_vec input; sigma_bar_v_hat_vec input; dp_hat_1 output
function dp_hat_1 = fcn(c3v, d_sigma_bar_v_vec, sigma_bar_v_hat_vec)
%%%% 计算扰动观测值dp_hat
iiuav = 1;
dp_hat_1 = d_sigma_bar_v_vec(:,iiuav) + c3v * sigma_bar_v_hat_vec(:,iiuav);

== matlab function sim_dist_pos_obs_paper/cal dp_hat agent 2 ==
  data: c3v input; d_sigma_bar_v_vec input; sigma_bar_v_hat_vec input; dp_hat_2 output
function dp_hat_2 = fcn(c3v, d_sigma_bar_v_vec, sigma_bar_v_hat_vec)
%%%% 计算扰动观测值dp_hat
iiuav = 2;
dp_hat_2 = d_sigma_bar_v_vec(:,iiuav) + c3v * sigma_bar_v_hat_vec(:,iiuav);

== matlab function sim_dist_pos_obs_paper/cal dp_hat agent 3 ==
  data: c3v input; d_sigma_bar_v_vec input; sigma_bar_v_hat_vec input; dp_hat_3 output
function dp_hat_3 = fcn(c3v, d_sigma_bar_v_vec, sigma_bar_v_hat_vec)
%%%% 计算扰动观测值dp_hat
iiuav = 3;
dp_hat_3 = d_sigma_bar_v_vec(:,iiuav) + c3v * sigma_bar_v_hat_vec(:,iiuav);

== matlab function sim_dist_pos_obs_paper/trans to column3 ==
  data: x input; y output
function y = fcn(x)
y = x(:);

== matlab function sim_dist_pos_obs_paper/cal dp_hat agent 4 ==
  data: c3v input; d_sigma_bar_v_vec input; sigma_bar_v_hat_vec input; dp_hat_4 output
function dp_hat_4 = fcn(c3v, d_sigma_bar_v_vec, sigma_bar_v_hat_vec)
%%%% 计算扰动观测值dp_hat
iiuav = 4;
dp_hat_4 = d_sigma_bar_v_vec(:,iiuav) + c3v * sigma_bar_v_hat_vec(:,iiuav);

== matlab function sim_dist_pos_obs_paper/cal dp_hat agent 5 ==
  data: c3v input; d_sigma_bar_v_vec input; sigma_bar_v_hat_vec input; dp_hat_5 output
function dp_hat_5 = fcn(c3v, d_sigma_bar_v_vec, sigma_bar_v_hat_vec)
%%%% 计算扰动观测值dp_hat
iiuav = 5;
dp_hat_5 = d_sigma_bar_v_vec(:,iiuav) + c3v * sigma_bar_v_hat_vec(:,iiuav);

== matlab function sim_dist_pos_obs_paper/combine dp_hat ==
  data: dp_hat_1 input; dp_hat_2 input; dp_hat_3 input; dp_hat_4 input; dp_hat_5 input; dp_hat_vec output
function dp_hat_vec  = fcn(dp_hat_1, dp_hat_2, dp_hat_3, dp_hat_4, dp_hat_5)
%%%% 合并扰动观测值dp_hat
dp_hat_vec = [dp_hat_1(:), dp_hat_2(:), dp_hat_3(:), dp_hat_4(:), dp_hat_5(:)];

== matlab function sim_dist_pos_obs_paper/cal abs 31 ==
  data: x input; y output
function y = fcn(x)
y = abs(x(:));

== matlab function sim_dist_pos_obs_paper/cal abs 32 ==
  data: x input; y output
function y = fcn(x)
y = abs(x(:));

== matlab function sim_dist_pos_obs_paper/cal theta_phi agent 1 ==
  data: alfa_theta input; phi_squ_1_1 input; theta_phi_1_1 output; phi_squ_2_1 input; phi_vec input; theta_phi_2_1 output
function [theta_phi_1_1, theta_phi_2_1] = fcn(alfa_theta, phi_squ_1_1, phi_squ_2_1, phi_vec)
%%%% 计算平滑递增函数
iiuav = 1;
theta_phi_1_1 = phi_squ_1_1(:) .* ( -1 + 2 ./ ( 1 + exp( -alfa_theta .* phi_vec(:,iiuav) ) ) );
theta_phi_2_1 = phi_squ_2_1(:) .* ( -1 + 2 ./ ( 1 + exp( -alfa_theta .* phi_vec(:,iiuav) ) ) );

== matlab function sim_dist_pos_obs_paper/choose ksi_est_err 31 ==
  data: x input; y output
function y = fcn(x)
iiuav = 1;
y = x(:,iiuav);

== matlab function sim_dist_pos_obs_paper/choose ksi_est_err 32 ==
  data: x input; y output
function y = fcn(x)
iiuav = 1;
y = x(:,iiuav);

== matlab function sim_dist_pos_obs_paper/cal abs 5 ==
  data: x input; y output
function y = fcn(x)
y = abs(x(:));

== matlab function sim_dist_pos_obs_paper/trans to column30 ==
  data: x input; y output
function y = fcn(x)
y = x(:);

== matlab function sim_dist_pos_obs_paper/trans to column31 ==
  data: x input; y output
function y = fcn(x)
y = x(:);

== matlab function sim_dist_pos_obs_paper/cal abs 33 ==
  data: x input; y output
function y = fcn(x)
y = abs(x(:));

== matlab function sim_dist_pos_obs_paper/cal abs 34 ==
  data: x input; y output
function y = fcn(x)
y = abs(x(:));

== matlab function sim_dist_pos_obs_paper/cal theta_phi agent 2 ==
  data: alfa_theta input; phi_squ_1_2 input; theta_phi_1_2 output; phi_squ_2_2 input; phi_vec input; theta_phi_2_2 output
function [theta_phi_1_2, theta_phi_2_2] = fcn(alfa_theta, phi_squ_1_2, phi_squ_2_2, phi_vec)
%%%% 计算平滑递增函数
iiuav = 2;
theta_phi_1_2 = phi_squ_1_2(:) .* ( -1 + 2 ./ ( 1 + exp( -alfa_theta .* phi_vec(:,iiuav) ) ) );
theta_phi_2_2 = phi_squ_2_2(:) .* ( -1 + 2 ./ ( 1 + exp( -alfa_theta .* phi_vec(:,iiuav) ) ) );

== matlab function sim_dist_pos_obs_paper/choose ksi_est_err 33 ==
  data: x input; y output
function y = fcn(x)
iiuav = 2;
y = x(:,iiuav);

== matlab function sim_dist_pos_obs_paper/choose ksi_est_err 34 ==
  data: x input; y output
function y = fcn(x)
iiuav = 2;
y = x(:,iiuav);

== matlab function sim_dist_pos_obs_paper/trans to column32 ==
  data: x input; y output
function y = fcn(x)
y = x(:);

== matlab function sim_dist_pos_obs_paper/trans to column33 ==
  data: x input; y output
function y = fcn(x)
y = x(:);

== matlab function sim_dist_pos_obs_paper/process velocity ==
  data: T0 input; T1 input; T2 input; PZ0 input; PZ1 input; R0 input; R1 input; Rx2 input; Ry2 input; Rz2 input; t input; V_init_out output
function V_init_out = fcn(T0, T1, T2, PZ0, PZ1, R0, R1, Rx2, Ry2, Rz2, t)
V_init_out = zeros(3, 1);
if t < T1 + 1e-05
    V_init_out(1, 1) = ( cos( ( 2 * pi * ( t - T0 ) ) / ( T0 - T1 ) ) * ( R0 - R1 ) ) / ( T0 - T1 ) ...
                                    - ( 2 * pi * sin( ( 2 * pi * ( t - T0 ) ) / ( T0 - T1 ) ) * ( R0 + ( ( R0 - R1 ) * ( t - T0 ) ) / ( T0 - T1 ) ) ) / ( T0 - T1 );
    V_init_out(2, 1) = ( sin( ( 2 * pi * ( t - T0 ) ) / ( T0 - T1 ) ) * ( R0 - R1 ) ) / ( T0 - T1 ) ...
                                    + ( 2 * pi * cos( ( 2 * pi * ( t - T0 ) ) / ( T0 - T1 ) ) * ( R0 + ( ( R0 - R1 ) * ( t - T0 ) ) / ( T0 - T1 ) ) ) / ( T0 - T1 );
    V_init_out(3, 1) = ( PZ0 - PZ1 ) / ( T0 - T1 );
else
    V_init_out(1, 1) = ( 2 * Rx2 * pi * sin( ( 2 * pi * ( t - T1 ) ) / ( T1 - T2 ) ) ) / ( T1 - T2 );
    V_init_out(2, 1) = ( 4 * Ry2 * pi * cos( ( 4 * pi * ( t - T1 ) ) / ( T1 - T2 ) ) ) / ( T1 - T2 );
    V_init_out(3, 1) = - ( 4 * Rz2 * pi * cos( ( 4 * pi * ( t - T1 ) ) / ( T1 - T2 ) ) ) / ( T1 - T2 );
end

== matlab function sim_dist_pos_obs_paper/cal abs 35 ==
  data: x input; y output
function y = fcn(x)
y = abs(x(:));

== matlab function sim_dist_pos_obs_paper/cal abs 36 ==
  data: x input; y output
function y = fcn(x)
y = abs(x(:));

== matlab function sim_dist_pos_obs_paper/cal theta_phi agent 3 ==
  data: alfa_theta input; phi_squ_1_3 input; theta_phi_1_3 output; phi_squ_2_3 input; phi_vec input; theta_phi_2_3 output
function [theta_phi_1_3, theta_phi_2_3] = fcn(alfa_theta, phi_squ_1_3, phi_squ_2_3, phi_vec)
%%%% 计算平滑递增函数
iiuav = 3;
theta_phi_1_3 = phi_squ_1_3(:) .* ( -1 + 2 ./ ( 1 + exp( -alfa_theta .* phi_vec(:,iiuav) ) ) );
theta_phi_2_3 = phi_squ_2_3(:) .* ( -1 + 2 ./ ( 1 + exp( -alfa_theta .* phi_vec(:,iiuav) ) ) );

== matlab function sim_dist_pos_obs_paper/choose ksi_est_err 35 ==
  data: x input; y output
function y = fcn(x)
iiuav = 3;
y = x(:,iiuav);

== matlab function sim_dist_pos_obs_paper/choose ksi_est_err 36 ==
  data: x input; y output
function y = fcn(x)
iiuav = 3;
y = x(:,iiuav);

== matlab function sim_dist_pos_obs_paper/trans to column34 ==
  data: x input; y output
function y = fcn(x)
y = x(:);

== matlab function sim_dist_pos_obs_paper/trans to column36 ==
  data: x input; y output
function y = fcn(x)
y = x(:);

== matlab function sim_dist_pos_obs_paper/cal abs 37 ==
  data: x input; y output
function y = fcn(x)
y = abs(x(:));

== matlab function sim_dist_pos_obs_paper/cal abs 38 ==
  data: x input; y output
function y = fcn(x)
y = abs(x(:));

== matlab function sim_dist_pos_obs_paper/cal theta_phi agent 4 ==
  data: alfa_theta input; phi_squ_1_4 input; theta_phi_1_4 output; phi_squ_2_4 input; phi_vec input; theta_phi_2_4 output
function [theta_phi_1_4, theta_phi_2_4] = fcn(alfa_theta, phi_squ_1_4, phi_squ_2_4, phi_vec)
%%%% 计算平滑递增函数
iiuav = 4;
theta_phi_1_4 = phi_squ_1_4(:) .* ( -1 + 2 ./ ( 1 + exp( -alfa_theta .* phi_vec(:,iiuav) ) ) );
theta_phi_2_4 = phi_squ_2_4(:) .* ( -1 + 2 ./ ( 1 + exp( -alfa_theta .* phi_vec(:,iiuav) ) ) );

== matlab function sim_dist_pos_obs_paper/choose ksi_est_err 37 ==
  data: x input; y output
function y = fcn(x)
iiuav = 4;
y = x(:,iiuav);

== matlab function sim_dist_pos_obs_paper/choose ksi_est_err 38 ==
  data: x input; y output
function y = fcn(x)
iiuav = 4;
y = x(:,iiuav);

== matlab function sim_dist_pos_obs_paper/trans to column37 ==
  data: x input; y output
function y = fcn(x)
y = x(:);

== matlab function sim_dist_pos_obs_paper/trans to column38 ==
  data: x input; y output
function y = fcn(x)
y = x(:);

== matlab function sim_dist_pos_obs_paper/cal abs 39 ==
  data: x input; y output
function y = fcn(x)
y = abs(x(:));

== matlab function sim_dist_pos_obs_paper/cal abs 40 ==
  data: x input; y output
function y = fcn(x)
y = abs(x(:));

== matlab function sim_dist_pos_obs_paper/cal theta_phi agent 5 ==
  data: alfa_theta input; phi_squ_1_5 input; theta_phi_1_5 output; phi_squ_2_5 input; phi_vec input; theta_phi_2_5 output
function [theta_phi_1_5, theta_phi_2_5] = fcn(alfa_theta, phi_squ_1_5, phi_squ_2_5, phi_vec)
%%%% 计算平滑递增函数
iiuav = 5;
theta_phi_1_5 = phi_squ_1_5(:) .* ( -1 + 2 ./ ( 1 + exp( -alfa_theta .* phi_vec(:,iiuav) ) ) );
theta_phi_2_5 = phi_squ_2_5(:) .* ( -1 + 2 ./ ( 1 + exp( -alfa_theta .* phi_vec(:,iiuav) ) ) );

== matlab function sim_dist_pos_obs_paper/choose ksi_est_err 39 ==
  data: x input; y output
function y = fcn(x)
iiuav = 5;
y = x(:,iiuav);

== matlab function sim_dist_pos_obs_paper/choose ksi_est_err 40 ==
  data: x input; y output
function y = fcn(x)
iiuav = 5;
y = x(:,iiuav);

== matlab function sim_dist_pos_obs_paper/trans to column39 ==
  data: x input; y output
function y = fcn(x)
y = x(:);

== matlab function sim_dist_pos_obs_paper/trans to column40 ==
  data: x input; y output
function y = fcn(x)
y = x(:);

== matlab function sim_dist_pos_obs_paper/combine theta_err_ksi1 ==
  data: theta_phi_1_1 input; theta_phi_1_2 input; theta_phi_1_3 input; theta_phi_1_4 input; theta_phi_1_5 input; theta_phi_1_vec output; theta_phi_2_1 input; theta_phi_2_vec output; theta_phi_2_2 input; theta_phi_2_3 input; theta_phi_2_4 input; theta_phi_2_5 input
function [theta_phi_1_vec, theta_phi_2_vec]  = fcn(theta_phi_1_1, theta_phi_1_2, theta_phi_1_3, theta_phi_1_4, theta_phi_1_5, ...
                                                                                            theta_phi_2_1, theta_phi_2_2, theta_phi_2_3, theta_phi_2_4, theta_phi_2_5)
%%%% 合并领导者位置观测器输出结果
theta_phi_1_vec = [theta_phi_1_1(:), theta_phi_1_2(:), theta_phi_1_3(:), theta_phi_1_4(:), theta_phi_1_5(:)];
theta_phi_2_vec = [theta_phi_2_1(:), theta_phi_2_2(:), theta_phi_2_3(:), theta_phi_2_4(:), theta_phi_2_5(:)];

== matlab function sim_dist_pos_obs_paper/desire formation position and velocity ==
  data: ksi0 input; eta0 input; delta_ksi_vec input; delta_eta_vec input; pos_i_des output; vel_i_des output
function [pos_i_des, vel_i_des] = fcn(ksi0, eta0, delta_ksi_vec, delta_eta_vec)
pos_i_des = zeros(3, 5);
vel_i_des = zeros(3, 5);
for iiuav = 1:5
    pos_i_des(:, iiuav) = ksi0(:) + delta_ksi_vec(:, iiuav);
    vel_i_des(:, iiuav) = eta0(:) + delta_eta_vec(:, iiuav);
end

== matlab function sim_dist_pos_obs_paper/cal ui agent 1 ==
  data: kai_u_1 input; ui_1 output; kai_u_2 input; d_chi_vec input; theta_phi_1_vec input; theta_phi_2_vec input; dp_hat_vec input
function ui_1 = fcn(kai_u_1, kai_u_2, d_chi_vec, theta_phi_1_vec, theta_phi_2_vec, dp_hat_vec)
%%%% 计算控制输入ui
iiuav = 1;
g0 = 9.80663;
e3 = [0;0;1];
ui_1 = g0 * e3 + d_chi_vec(:,iiuav) - kai_u_1 * theta_phi_1_vec(:,iiuav) - kai_u_2 * theta_phi_2_vec(:,iiuav) - dp_hat_vec(:,iiuav);

== matlab function sim_dist_pos_obs_paper/cal ui agent 2 ==
  data: kai_u_1 input; ui_2 output; kai_u_2 input; d_chi_vec input; theta_phi_1_vec input; theta_phi_2_vec input; dp_hat_vec input
function ui_2 = fcn(kai_u_1, kai_u_2, d_chi_vec, theta_phi_1_vec, theta_phi_2_vec, dp_hat_vec)
%%%% 计算控制输入ui
iiuav = 2;
g0 = 9.80663;
e3 = [0;0;1];
ui_2 = g0 * e3 + d_chi_vec(:,iiuav) - kai_u_1 * theta_phi_1_vec(:,iiuav) - kai_u_2 * theta_phi_2_vec(:,iiuav) - dp_hat_vec(:,iiuav);

== matlab function sim_dist_pos_obs_paper/cal ui agent 3 ==
  data: kai_u_1 input; ui_3 output; kai_u_2 input; d_chi_vec input; theta_phi_1_vec input; theta_phi_2_vec input; dp_hat_vec input
function ui_3 = fcn(kai_u_1, kai_u_2, d_chi_vec, theta_phi_1_vec, theta_phi_2_vec, dp_hat_vec)
%%%% 计算控制输入ui
iiuav = 3;
g0 = 9.80663;
e3 = [0;0;1];
ui_3 = g0 * e3 + d_chi_vec(:,iiuav) - kai_u_1 * theta_phi_1_vec(:,iiuav) - kai_u_2 * theta_phi_2_vec(:,iiuav) - dp_hat_vec(:,iiuav);

== matlab function sim_dist_pos_obs_paper/cal ui agent 4 ==
  data: kai_u_1 input; ui_4 output; kai_u_2 input; d_chi_vec input; theta_phi_1_vec input; theta_phi_2_vec input; dp_hat_vec input
function ui_4 = fcn(kai_u_1, kai_u_2, d_chi_vec, theta_phi_1_vec, theta_phi_2_vec, dp_hat_vec)
%%%% 计算控制输入ui
iiuav = 4;
g0 = 9.80663;
e3 = [0;0;1];
ui_4 = g0 * e3 + d_chi_vec(:,iiuav) - kai_u_1 * theta_phi_1_vec(:,iiuav) - kai_u_2 * theta_phi_2_vec(:,iiuav) - dp_hat_vec(:,iiuav);

== matlab function sim_dist_pos_obs_paper/cal ui agent 5 ==
  data: kai_u_1 input; ui_5 output; kai_u_2 input; d_chi_vec input; theta_phi_1_vec input; theta_phi_2_vec input; dp_hat_vec input
function ui_5 = fcn(kai_u_1, kai_u_2, d_chi_vec, theta_phi_1_vec, theta_phi_2_vec, dp_hat_vec)
%%%% 计算控制输入ui
iiuav = 5;
g0 = 9.80663;
e3 = [0;0;1];
ui_5 = g0 * e3 + d_chi_vec(:,iiuav) - kai_u_1 * theta_phi_1_vec(:,iiuav) - kai_u_2 * theta_phi_2_vec(:,iiuav) - dp_hat_vec(:,iiuav);

== matlab function sim_dist_pos_obs_paper/combine ui ==
  data: ui_1 input; ui_2 input; ui_3 input; ui_4 input; ui_5 input; ui output
function ui  = fcn(ui_1, ui_2, ui_3, ui_4, ui_5)
%%%% 合并控制输入ui
ui = [ui_1(:), ui_2(:), ui_3(:), ui_4(:), ui_5(:)];

== matlab function sim_dist_pos_obs_paper/cal disturbance observation error dp_tilt ==
  data: dp_vec input; dp_tilt_vec output; dp_hat_vec input
function dp_tilt_vec = fcn(dp_vec, dp_hat_vec)
%%%% 计算扰动观测器估计误差dp_tilt
dp_tilt_vec = zeros(3,5);
for iiuav = 1:5
    dp_tilt_vec(:,iiuav) = dp_vec(:,iiuav) - dp_hat_vec(:,iiuav);
end

== matlab function sim_dist_pos_obs_paper/choose dp_tilt_1 ==
  data: x input; y output
function y = fcn(x)
iiuav = 1;
y = x(:,iiuav);

== matlab function sim_dist_pos_obs_paper/choose dp_tilt_2 ==
  data: x input; y output
function y = fcn(x)
iiuav = 2;
y = x(:,iiuav);

== matlab function sim_dist_pos_obs_paper/choose dp_tilt_3 ==
  data: x input; y output
function y = fcn(x)
iiuav = 3;
y = x(:,iiuav);

== matlab function sim_dist_pos_obs_paper/choose dp_tilt_4 ==
  data: x input; y output
function y = fcn(x)
iiuav = 4;
y = x(:,iiuav);
